simulink model "PV_new"  (R2015a)
settings: Solver=ode45  StartTime=0.0  StopTime=10.0  RelTol=1e-3
values from neighbouring files (symbols this model uses):
  k = 1.3806e-23    [sunpower305.m]
  q = 1.6022e-19    [sunpower305.m]
  Rp = 993.51    [sunpower305.m]
  Rs = 0.037998    [sunpower305.m]
  T = 273+25    (= 298)    [sunpower305.m]
undefined symbols (not defined in the file or in its folder): a, G, Gn, I, Ipvn, Iscn, Ki, Kv, Npp, Ns, Nss, Tn, V, Vocn
libraries: powerlib x7, simulink x2
settings Model: Creator=Limon  LastModifiedBy=Limon

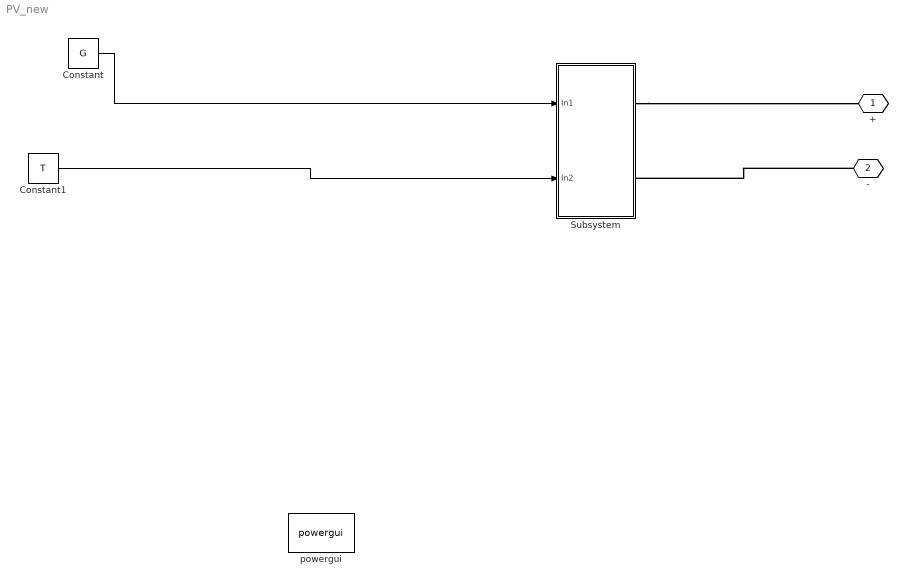
== system PV_new ==
  Constant : Constant  Value=G
  Constant1 : Constant  Value=T
  Subsystem : Subsystem
  powergui : powerlib/powergui  Priority=1  SimulationMode=Discrete  SolverType=Tustin/Backward Euler (TBE)  SampleTime=1e-3  frequency=60  SPID=off  DisableSnubberDevices=off  DisableRonSwitches=off  DisableVfSwitches=off  SwTol=0  DisplayEquations=off  Interpol=off  methode=off  Ts=100  FunctionMessages=off  echomessages=off  HookPort=off  EnableUseOfTLC=off  x0status=blocks  frequencyindice=0  Pbase=100e6  ErrMax=1e-4  Iterations=50  UnitsV=kV  UnitsW=MW  buscounter=0  RestoreLinks=warning  ResistiveCurrentMeasurement=off  Frange=[0:2:500]  Ylog=off  Xlog=on  ShowGrid=off  save=off  variable=ZData  structure=0  ZoomFFT=off  StartTime=0.0  cycles=1  DisplayStyle=1  fundamental=60  FreqAxis=off  MaxFrequency=1000  frequencyindicesteady=1  RmsSteady=1  display=off
  + : PMIOPort  Tag=PMCPort  Port=1  Side=Left
  - : PMIOPort  Tag=PMCPort  Port=2  Side=Right
  wires:
  Constant/1 -> Subsystem/1(In1)
  Constant1/1 -> Subsystem/2(In2)
  connections:
  Subsystem/RConn1 -- +/RConn1
  -/RConn1 -- Subsystem/RConn2

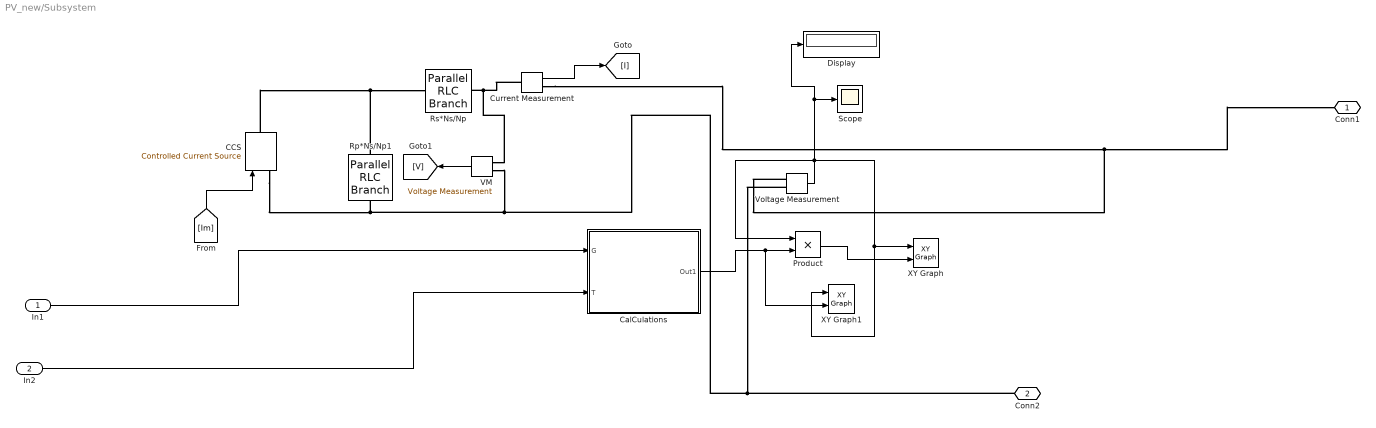
== system PV_new/Subsystem ==
  In1 : Inport
  In2 : Inport  Port=2
  CCS : powerlib/Electrical Sources/Controlled Current Source  Initialize=on  Source_Type=AC  Amplitude=0  Phase=0  Frequency=0  Measurements=None
  CalCulations : Subsystem
  Current Measurement : powerlib/Measurements/Current Measurement  PhasorSimulation=off  OutputType=Complex  PSBequivalent=0
  Display : Display
  Product : Product
  Rp*Ns/Np1 : powerlib/Elements/Parallel RLC Branch  LConnTagsString=a  RConnTagsString=__new0  BranchType=R  Resistance=Rp*Nss/Npp  Inductance=1e-3  SetiL0=off  InitialCurrent=0  Capacitance=1e-6  Setx0=off  InitialVoltage=0  Measurements=None
  Rs*Ns/Np : powerlib/Elements/Parallel RLC Branch  LConnTagsString=a  RConnTagsString=__new0  BranchType=R  Resistance=Rs*Nss/Npp  Inductance=1e-3  SetiL0=off  InitialCurrent=0  Capacitance=1e-6  Setx0=off  InitialVoltage=0  Measurements=None
  Scope : Scope
  VM : powerlib/Measurements/Voltage Measurement  PhasorSimulation=off  OutputType=Complex  PSBequivalent=0
  Voltage Measurement : powerlib/Measurements/Voltage Measurement  PhasorSimulation=off  OutputType=Complex  PSBequivalent=0
  XY Graph : simulink/Sinks/XY Graph  xmin=0  xmax=30  ymin=0  ymax=60  st=-1
  XY Graph1 : simulink/Sinks/XY Graph  xmin=0  xmax=30  ymin=0  ymax=5  st=-1
  Conn1 : PMIOPort  Port=1  Side=Right
  Conn2 : PMIOPort  Port=2  Side=Right
  wires:
  CalCulations/1(Out1) -> XY Graph1/2, Product/2
  In1/1 -> CalCulations/1(G)
  In2/1 -> CalCulations/2(T)
  Voltage Measurement/1 -> XY Graph1/1, XY Graph/1, Product/1, Scope/1, Display/1
  Product/1 -> XY Graph/2
  [Im] -> CCS/1
  VM/1 -> [V]
  Current Measurement/1 -> [I]
  connections:
  Voltage Measurement/LConn1 -- Conn1/RConn1 -- Current Measurement/RConn1
  Voltage Measurement/LConn2 -- Conn2/RConn1 -- CCS/LConn1 -- Rp*Ns/Np1/RConn1 -- VM/LConn1
  Current Measurement/LConn1 -- VM/LConn2 -- Rs*Ns/Np/RConn1
  Rp*Ns/Np1/LConn1 -- Rs*Ns/Np/LConn1 -- CCS/RConn1

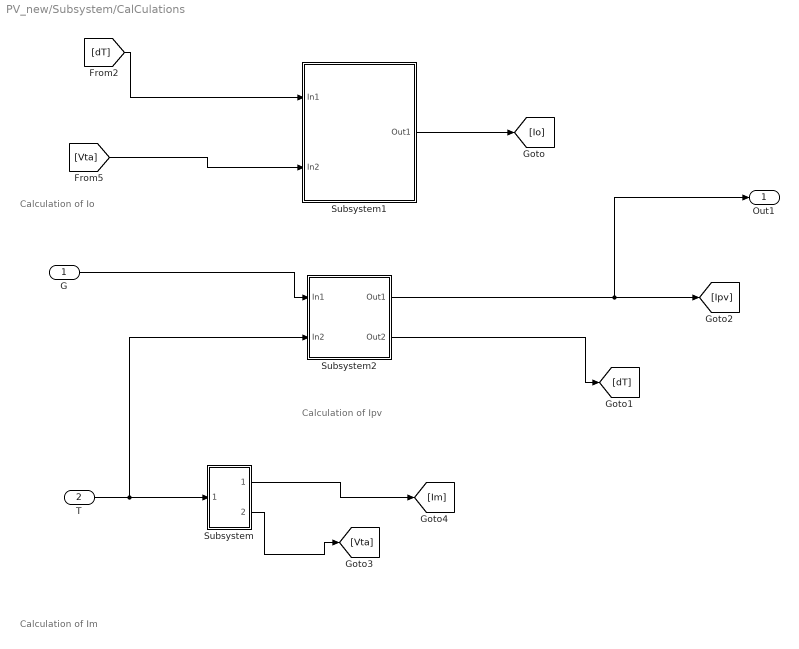
== system PV_new/Subsystem/CalCulations ==
  note: Calculation of Ipv
  note: Calculation of Im
  note: Calculation of Io
  G : Inport
  T : Inport  Port=2
  Subsystem : Subsystem
  Subsystem1 : Subsystem
  Subsystem2 : Subsystem
  Out1 : Outport
  wires:
  T/1 -> Subsystem2/2(In2), Subsystem/1(In1)
  [Vta] -> Subsystem1/2(In2)
  Subsystem2/2(Out2) -> [dT]
  G/1 -> Subsystem2/1(In1)
  Subsystem/2(Out2) -> [Vta]
  Subsystem/1(Out1) -> [Im]
  Subsystem2/1(Out1) -> Out1/1, [Ipv]
  [dT] -> Subsystem1/1(In1)
  Subsystem1/1(Out1) -> [Io]

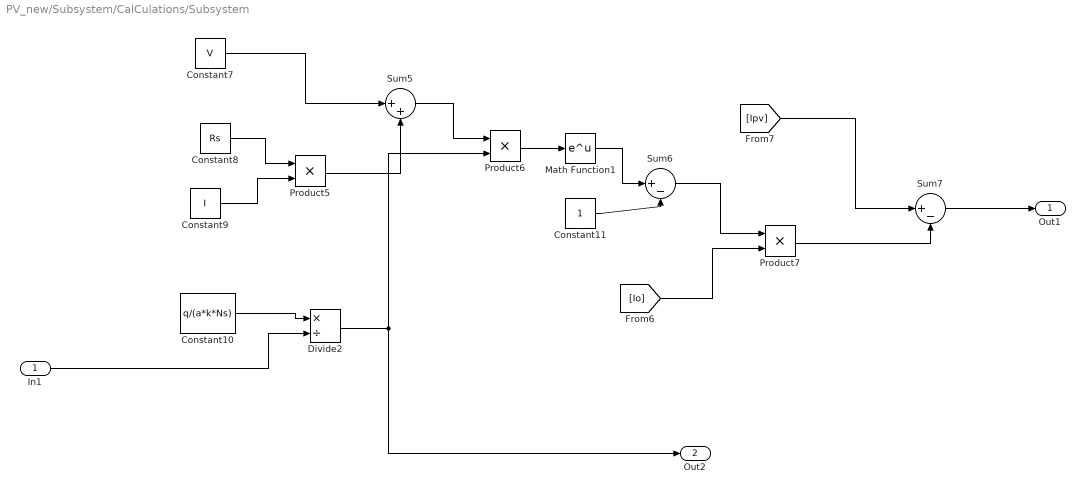
== system PV_new/Subsystem/CalCulations/Subsystem ==
  In1 : Inport
  Constant10 : Constant  Value=q/(a*k*Ns)
  Constant11 : Constant
  Constant7 : Constant  Value=V
  Constant8 : Constant  Value=Rs
  Constant9 : Constant  Value=I
  Divide2 : Product  Inputs=*/
  Math Function1 : Math  SaturateOnIntegerOverflow=on
  Product5 : Product
  Product6 : Product
  Product7 : Product
  Sum5 : Sum  Inputs=|++
  Sum6 : Sum  Inputs=|+-
  Sum7 : Sum  Inputs=|+-
  Out1 : Outport
  Out2 : Outport  Port=2
  wires:
  Product6/1 -> Math Function1/1
  Divide2/1 -> Out2/1, Product6/2
  Constant10/1 -> Divide2/1
  [Ipv] -> Sum7/1
  [Io] -> Product7/2
  Constant8/1 -> Product5/1
  Product7/1 -> Sum7/2
  Constant11/1 -> Sum6/2
  In1/1 -> Divide2/2
  Product5/1 -> Sum5/2
  Sum7/1 -> Out1/1
  Constant7/1 -> Sum5/1
  Constant9/1 -> Product5/2
  Sum5/1 -> Product6/1
  Sum6/1 -> Product7/1
  Math Function1/1 -> Sum6/1

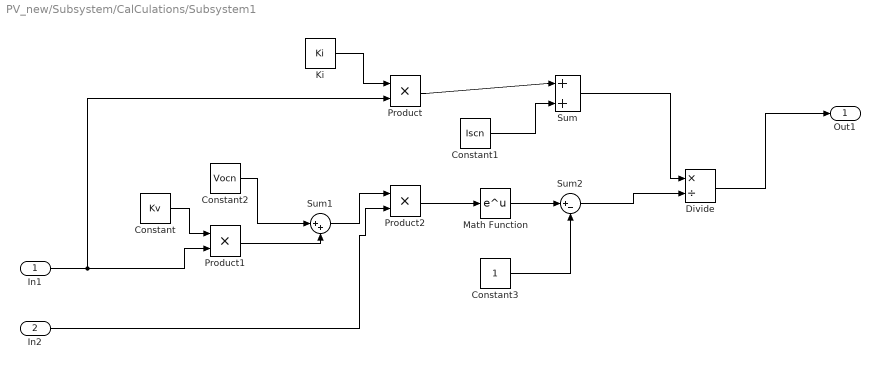
== system PV_new/Subsystem/CalCulations/Subsystem1 ==
  In1 : Inport
  In2 : Inport  Port=2
  Constant : Constant  Value=Kv
  Constant1 : Constant  Value=Iscn
  Constant2 : Constant  Value=Vocn
  Constant3 : Constant
  Divide : Product  Inputs=*/
  Ki : Constant  Value=Ki
  Math Function : Math  SaturateOnIntegerOverflow=on
  Product : Product
  Product1 : Product
  Product2 : Product
  Sum : Sum  Inputs=|++
  Sum1 : Sum  Inputs=|++
  Sum2 : Sum  Inputs=|+-
  Out1 : Outport
  wires:
  Product2/1 -> Math Function/1
  Math Function/1 -> Sum2/1
  Ki/1 -> Product/1
  Sum/1 -> Divide/1
  Constant3/1 -> Sum2/2
  Sum2/1 -> Divide/2
  Constant1/1 -> Sum/2
  Product1/1 -> Sum1/2
  In2/1 -> Product2/2
  Sum1/1 -> Product2/1
  Constant2/1 -> Sum1/1
  Constant/1 -> Product1/1
  Divide/1 -> Out1/1
  Product/1 -> Sum/1
  In1/1 -> Product/2, Product1/2

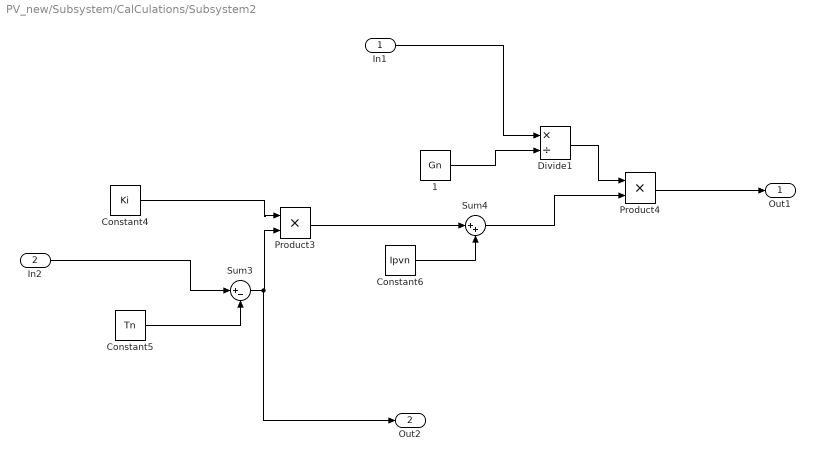
== system PV_new/Subsystem/CalCulations/Subsystem2 ==
  In1 : Inport
  In2 : Inport  Port=2
  1 : Constant  Value=Gn
  Constant4 : Constant  Value=Ki
  Constant5 : Constant  Value=Tn
  Constant6 : Constant  Value=Ipvn
  Divide1 : Product  Inputs=*/
  Product3 : Product
  Product4 : Product
  Sum3 : Sum  Inputs=|+-
  Sum4 : Sum  Inputs=|++
  Out1 : Outport
  Out2 : Outport  Port=2
  wires:
  Product4/1 -> Out1/1
  Sum3/1 -> Out2/1, Product3/2
  In1/1 -> Divide1/1
  1/1 -> Divide1/2
  In2/1 -> Sum3/1
  Constant5/1 -> Sum3/2
  Constant6/1 -> Sum4/2
  Product3/1 -> Sum4/1
  Sum4/1 -> Product4/2
  Constant4/1 -> Product3/1
  Divide1/1 -> Product4/1
